simulink model "observador"  (R2022b)
settings: Solver=VariableStepAuto  StartTime=0.0  StopTime=30  RelTol=1e-3
values from neighbouring files (symbols this model uses):
  disturbio = 0.24    [lab12.m]
  R = 1.18    [lab12.m]
  sistema_inicial = [-0.11; -0.11]    [lab12.m]
undefined symbols (not defined in the file or in its folder): Ac, Bc, Cc, Dc
settings Model: Creator=mathe  LastModifiedBy=mathe

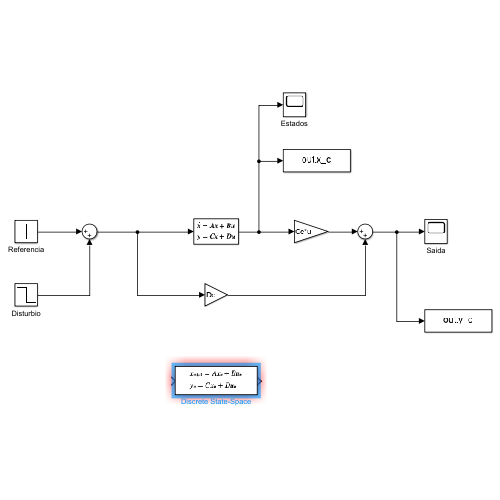
[thumbnail: Simulink's stored preview of the top-level diagram]
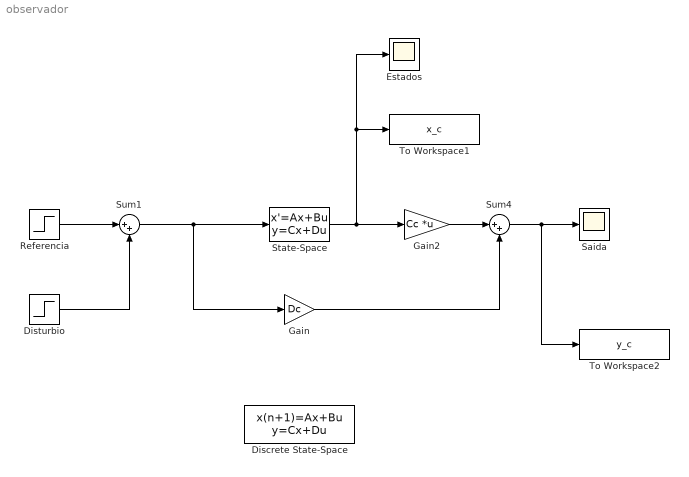
== system observador ==
  Discrete State-Space : DiscreteStateSpace  A=Ac  B=Bc  C=[1 0; 0 1]  D=[0; 0]  InitialCondition=sistema_inicial  SampleTime=0.4855
  Disturbio : Step  Time=15  After=disturbio  SampleTime=0
  Estados : Scope
  Gain : Gain  Gain=Dc
  Gain2 : Gain  Gain=Cc  Multiplication=Matrix(K*u)
  Referencia : Step  Time=0  After=R  SampleTime=0
  Saida : Scope
  State-Space : StateSpace  A=Ac  B=Bc  C=[1 0; 0 1]  D=[0; 0]  InitialCondition=0
  Sum1 : Sum  Inputs=|++
  Sum4 : Sum  Inputs=|++
  To Workspace1 : ToWorkspace  VariableName=x_c  SaveFormat=Timeseries  SampleTime=-1
  To Workspace2 : ToWorkspace  VariableName=y_c  SaveFormat=Timeseries  SampleTime=-1
  wires:
  State-Space/1 -> Gain2/1, Estados/1, To Workspace1/1
  Sum4/1 -> To Workspace2/1, Saida/1
  Sum1/1 -> State-Space/1, Gain/1
  Referencia/1 -> Sum1/1
  Disturbio/1 -> Sum1/2
  Gain2/1 -> Sum4/1
  Gain/1 -> Sum4/2
